simulink model "model"  (R2013b)
settings: Solver=ode45  StartTime=0.0  StopTime=50  MaxStep=0.01  RelTol=1e-3
undefined symbols (not defined in the file or in its folder): A, n, ref, temp_0
libraries: powerlib_meascontrol x1, dspmtrx3 x1
settings Model: Creator=Marta_2805  LastModifiedBy=Marta_2805
settings SolverCC: AutoInsertRateTranBlk=on

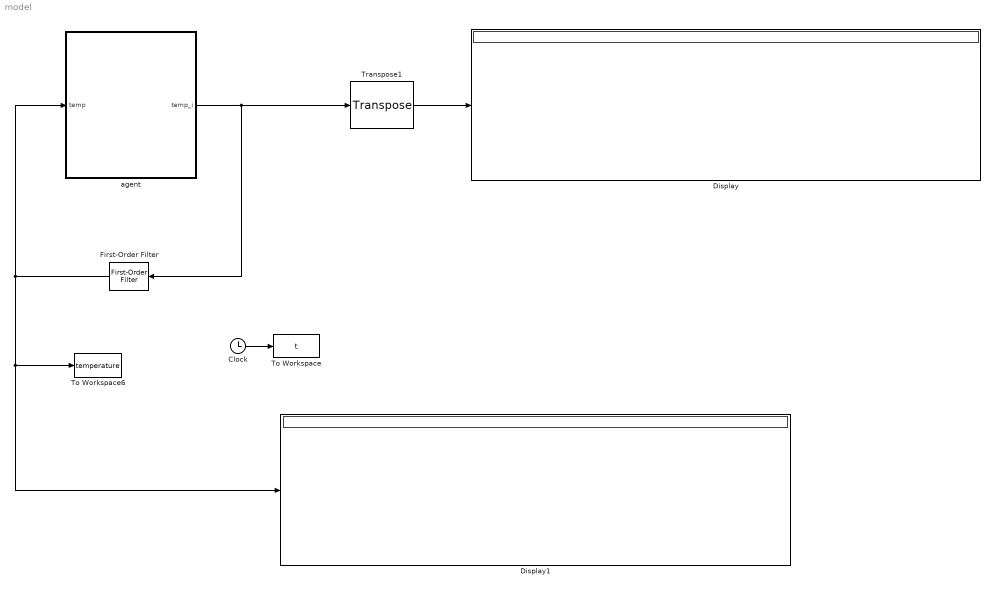
== system model ==
  Clock : Clock
  Display : Display
  Display1 : Display
  First-Order Filter : powerlib_meascontrol/Filters/First-Order Filter  FilterType=Lowpass  Tc=1  Ts=0  Initialize=on  Vac_Init=[0, 0, 60]  Vdc_Init=0  PlotResponse=off  FreqRange="[0,  200,  1]"
  To Workspace : ToWorkspace  VariableName=t  SampleTime=-1
  To Workspace6 : ToWorkspace  VariableName=temperature  SampleTime=-1
  Transpose1 : dspmtrx3/Transpose  Hermitian=off  overflowFlag=off
  "agent " : Subsystem
  wires:
  "agent "/1(temp_i) -> First-Order Filter/1, Transpose1/1
  Transpose1/1 -> Display/1
  Clock/1 -> To Workspace/1
  First-Order Filter/1 -> To Workspace6/1, Display1/1, "agent "/1(temp)

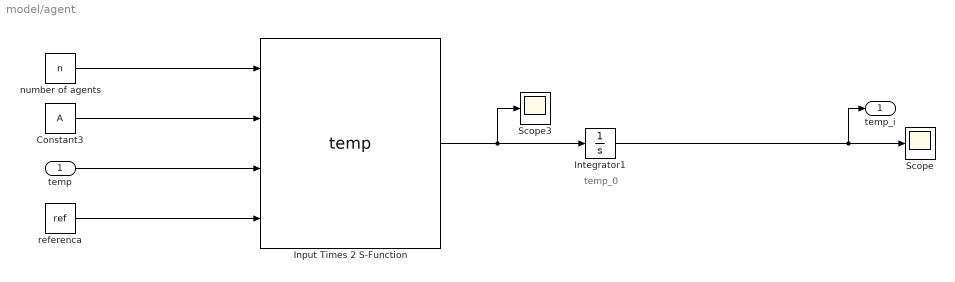
== system model/agent  ==
  note: temp_0
  temp : Inport
  Constant3 : Constant  Value=A
  Input Times 2 S-Function : S-Function  FunctionName=temp  EnableBusSupport=off
  Integrator1 : Integrator  InitialCondition=temp_0
  Scope : Scope
      settings: TimeRange=20  YMin=0.25  YMax=0.95
  Scope3 : Scope
      settings: TimeRange=20  YMin=0.25  YMax=0.95  SaveName=ScopeData3
  number of agents : Constant  Value=n
  referenca : Constant  Value=ref
  temp_i : Outport
  wires:
  Input Times 2 S-Function/1 -> Scope3/1, Integrator1/1
  number of agents/1 -> Input Times 2 S-Function/1
  Constant3/1 -> Input Times 2 S-Function/2
  temp/1 -> Input Times 2 S-Function/3
  Integrator1/1 -> temp_i/1, Scope/1
  referenca/1 -> Input Times 2 S-Function/4
